simulink model "model2"  (R2022a)
settings: Solver=VariableStepAuto  StartTime=0.0  StopTime=1000  RelTol=1e-3
values from neighbouring files (symbols this model uses):
  A = [   0    1 ... (first row only)    [config.m]
  A_m = [     0      1 ... (first row only)    [config.m]
  b = [0 ... (first row only)    [config.m]
  b_m = [0 ... (first row only)    [config.m]
  disturbance = 0    [config.m]    (also in task1.m = 1; task2.m = 1)
  gamma = 10000    [task1.m]    (also in task2.m = 100)
  k = b_0/a_m_0    (= 0.0434782608696)    [config.m]
  P = lyap(A_m', Q)    [config.m]
  sigma = 10    [task1.m]    (also in task2.m)
  x_0 = [1; 0]    [config.m]
settings Model: Creator=Vvlad  LastModifiedBy=Vvlad

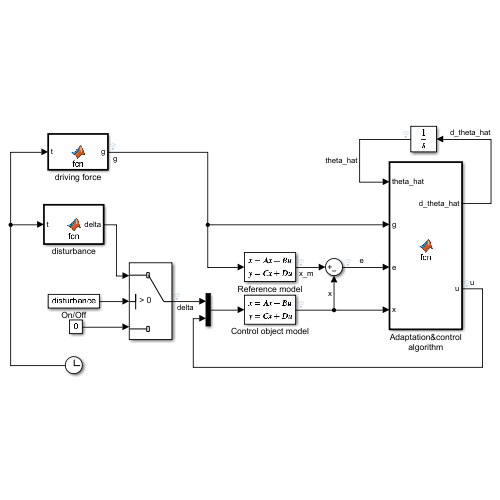
[thumbnail: Simulink's stored preview of the top-level diagram]
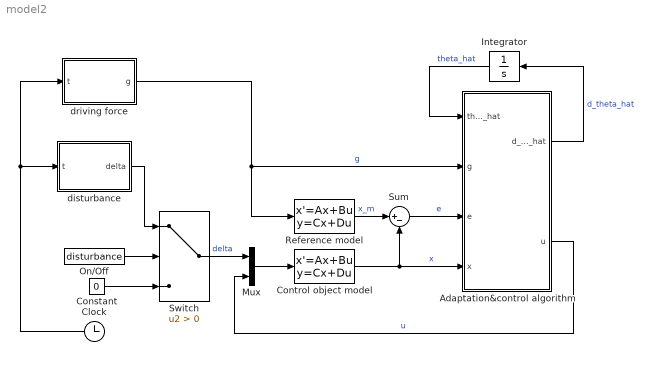
== system model2 ==
  Adaptation&control algorithm : MATLAB Function  TreatAsAtomicUnit=on
  Clock : Clock
  Constant : Constant  Value=0
  Control object model : StateSpace  A=A  B=[eye(2) b]  C=eye(2)  D=zeros(2,3)  InitialCondition=x_0
  Integrator : Integrator
  Mux : Mux  Inputs=2
  On/Off : Constant  Value=disturbance
  Reference model : StateSpace  A=A_m  B=b_m  C=eye(2)  D=[0;0]  InitialCondition=0
  Sum : Sum  Inputs=|+-
  Switch : Switch  Criteria=u2 > Threshold  SaturateOnIntegerOverflow=off  InputSameDT=off
  disturbance : MATLAB Function  TreatAsAtomicUnit=on
  driving force : MATLAB Function  TreatAsAtomicUnit=on
  wires:
  Clock/1 -> driving force/1(t), disturbance/1(t)
  driving force/1(g) -> Adaptation&control algorithm/2(g), Reference model/1  "g"
  Control object model/1 -> Sum/2, Adaptation&control algorithm/4(x)  "x"
  Sum/1 -> Adaptation&control algorithm/3(e)  "e"
  Adaptation&control algorithm/2(u) -> Mux/2  "u"
  Reference model/1 -> Sum/1  "x_m"
  Mux/1 -> Control object model/1
  disturbance/1(delta) -> Switch/1
  Adaptation&control algorithm/1(d_theta_hat) -> Integrator/1  "d_theta_hat"
  Integrator/1 -> Adaptation&control algorithm/1(theta_hat)  "theta_hat"
  On/Off/1 -> Switch/2
  Constant/1 -> Switch/3
  Switch/1 -> Mux/1  "delta"

== matlab function model2/driving force ==
  data: t input; g output
function g = fcn(t)

g = 2*sign(sin(0.4*t)) + 3;

== matlab function model2/disturbance ==
  data: t input; delta output
function delta = fcn(t)

delta = [0.6*sin(10*t) + 0.1*sin(50*t);
        0.5*cos(12*t) + 0.2*sin(30*t)];

== matlab function model2/Adaptation&control algorithm ==
  data: theta_hat input; d_theta_hat output; g input; e input; x input; u output; gamma parameter; b parameter; P parameter; k parameter; sigma parameter
function [d_theta_hat, u]  = fcn(theta_hat, g, e, x, gamma, b, P, k, sigma)

d_theta_hat = -sigma*theta_hat + gamma*x*b'*P*e;
u = theta_hat'*x + 1/k*g;
